simulink subsystem "OdometriaWilly"  (R2021b)
settings: Solver=VariableStepAuto  StartTime=0.0  StopTime=10.0  RelTol=1e-3
undefined symbols (not defined in the file or in its folder): DiscIntNeverNeededParam
settings Model: Creator=Mauri  LastModifiedBy=Mauri

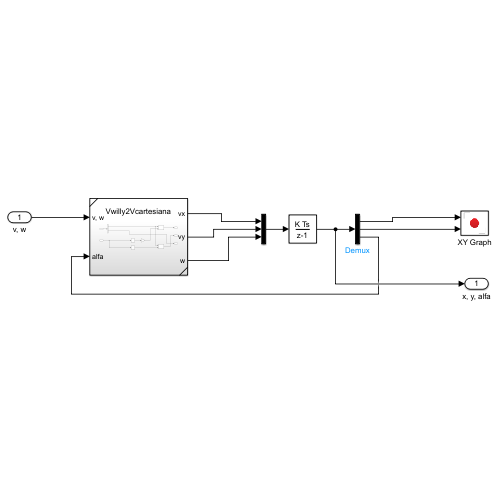
[thumbnail: Simulink's stored preview of the top-level diagram]
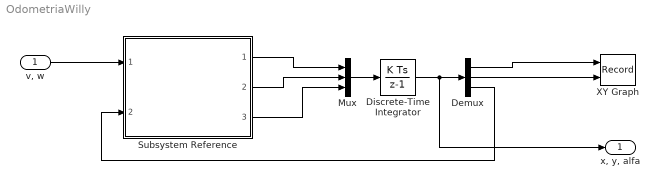
== system OdometriaWilly ==
  "v, w" : Inport
  Demux : Demux  Outputs=3
  Discrete-Time Integrator : DiscreteIntegrator  SampleTime=-1  ICPrevOutput=DiscIntNeverNeededParam  ICPrevScaledInput=DiscIntNeverNeededParam
  Mux : Mux  Inputs=3
  Subsystem Reference : Subsystem  ReferencedSubsystem=Vwilly2Vcartesiana
  XY Graph : Record  FileSettingsInternal="{\"entries\":[{\"content\":{\"excelSettings\":{\"content\":{},\"type\":\"Streamout.ExcelSettings\"}},\"type\":\"Streamout.FileSettingStorage\",\"uuid\":\"67e2448d-059d-483c-b416-7bb3546c2b38\"}],\"packageUris\":[\"http://schema.mathworks.com/mf0/streamout_blocks/R2020a\"],\"version\":\"1.0\"}"  Layout=[1 1]  SignalsInternal="{\"entries\":[{\"content\":{\"signals\":[{\"content\":{\"blockPath\":[\"untitled/XY Graph\"],\"channel\":[],\"dimensions\":[1],\"domain\":\"untitled/XY Graph\",\"lineColor\":\"#a2142f\",\"plots\":[1],\"port\":1,\"sid\":[],\"signalID\":13648,\"signalName\":\"XY Graph:1\"},\"type\":\"RecordBlkView.Signal\",\"uuid\":\"b70b9bfa-4167-4a2e-a278-4803edb2af31\"},{\"content\":{\"blockPath\":[\"untitled/XY Graph\"],\"channel\":[],\"dimensions\":[1],\"domain\":\"untitled/XY Graph\",\"lineColor\":\"#139fff\",\"plots\":[1],\"port\":2,\"sid\":[],\"signalID\":13651,\"signalName\":\"XY Graph:2\"},\"type\":\"RecordBlkView.Signal\",\"uuid\":\"62fbbcd6-2804-42b9-83de-03ea2f53de04\"}]},\"type\":\"RecordBlkView.InputSignals\",\"uuid\":\"e992c8d7-0512-4398-a6fc-20f6192cdc90\"}],\"packageUris\":[\"http://schema.mathworks.com/mf0/streamout_blocks/R2020a\"],\"version\":\"1.0\"}"  VisualizationBindings="{\"xyplotplugin\":{\"info\":[{\"series\":[{\"bindingParametersList\":[{\"parameter\":\"X-Axis\",\"signalID\":13648,\"signalName\":\"XY Graph:1\"},{\"parameter\":\"Y-Axis\",\"signalID\":13651,\"signalName\":\"XY Graph:2\"}],\"seriesID\":28241}],\"subplotID\":1}]}}"  CompatibilityTag=XY
  "x, y, alfa" : Outport
  wires:
  Subsystem Reference/1 -> Mux/1
  Subsystem Reference/2 -> Mux/2
  Subsystem Reference/3 -> Mux/3
  Mux/1 -> Discrete-Time Integrator/1
  Discrete-Time Integrator/1 -> "x, y, alfa"/1, Demux/1
  Demux/3 -> Subsystem Reference/2
  Demux/1 -> XY Graph/1
  Demux/2 -> XY Graph/2
  "v, w"/1 -> Subsystem Reference/1
